simulink model "MotoSimpleECU"  (R2026b)
settings: Solver=VariableStepAuto
undefined symbols (not defined in the file): CtrlEcuRevLim, DiscIntNeverNeededParam, PlntEngTqMax
libraries: simulink x1
settings Model: Creator=The MathWorks, Inc.  LastModifiedBy=The MathWorks, Inc.

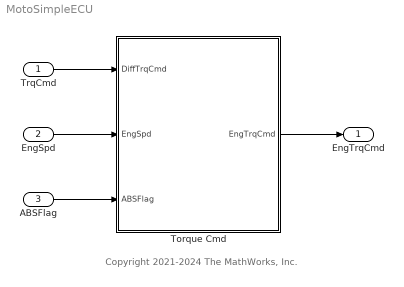
== system MotoSimpleECU ==
  note: Copyright 2021-2024 The MathWorks, Inc.
  TrqCmd : Inport
  EngSpd : Inport  Port=2
  ABSFlag : Inport  Port=3
  Torque Cmd : Subsystem  TreatAsAtomicUnit=on  SystemSampleTime=.01
  EngTrqCmd : Outport  VectorParamsAs1DForOutWhenUnconnected=off
  wires:
  ABSFlag/1 -> Torque Cmd/3(ABSFlag)
  Torque Cmd/1(EngTrqCmd) -> EngTrqCmd/1
  TrqCmd/1 -> Torque Cmd/1(DiffTrqCmd)
  EngSpd/1 -> Torque Cmd/2(EngSpd)

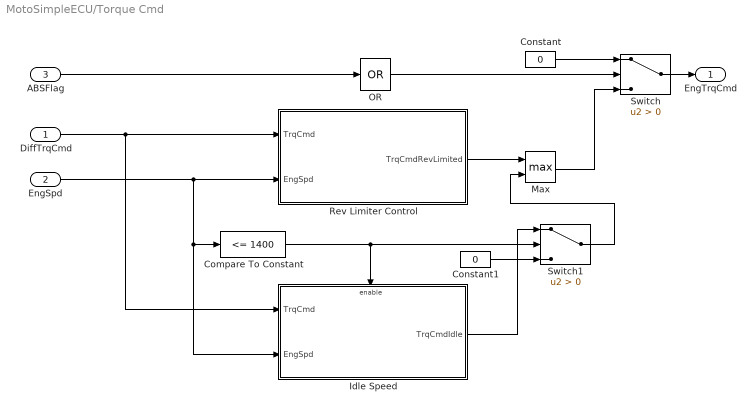
== system MotoSimpleECU/Torque Cmd ==
  DiffTrqCmd : Inport
  EngSpd : Inport  Port=2  Unit=rpm
  ABSFlag : Inport  Port=3
  Compare To Constant : simulink/Logic and Bit Operations/Compare To Constant  relop=<=  const=1400  OutDataTypeStr=boolean  ZeroCross=off
  Constant : Constant  Value=0
  Constant1 : Constant  Value=0
  Idle Speed : Subsystem
  Max : MinMax  Function=max  Inputs=2
  OR : Logic  Operator=OR  Inputs=1  AllPortsSameDT=off  OutDataTypeStr=boolean
  Rev Limiter Control : Subsystem
  Switch : Switch  Criteria=u2 > Threshold  ZeroCross=off  SaturateOnIntegerOverflow=off  InputSameDT=off
  Switch1 : Switch  Criteria=u2 > Threshold  ZeroCross=off  SaturateOnIntegerOverflow=off  InputSameDT=off
  EngTrqCmd : Outport
  wires:
  Switch1/1 -> Max/2
  Constant1/1 -> Switch1/3
  Compare To Constant/1 -> Switch1/2, Idle Speed/Enable
  Idle Speed/1(TrqCmdIdle) -> Switch1/1
  Rev Limiter Control/1(TrqCmdRevLimited) -> Max/1
  DiffTrqCmd/1 -> Rev Limiter Control/1(TrqCmd), Idle Speed/1(TrqCmd)
  EngSpd/1 -> Rev Limiter Control/2(EngSpd), Compare To Constant/1, Idle Speed/2(EngSpd)
  Max/1 -> Switch/3
  Switch/1 -> EngTrqCmd/1
  ABSFlag/1 -> OR/1
  Constant/1 -> Switch/1
  OR/1 -> Switch/2

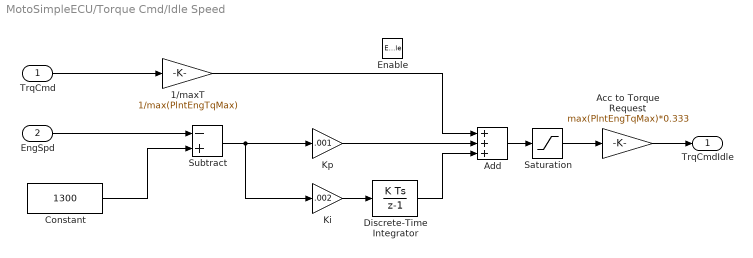
== system MotoSimpleECU/Torque Cmd/Idle Speed ==
  TrqCmd : Inport
  EngSpd : Inport  Port=2
  Enable : EnablePort  StatesWhenEnabling=reset  ZeroCross=off
  1/maxT : Gain  Gain=1/max(PlntEngTqMax)
  Acc to Torque Request : Gain  Gain=max(PlntEngTqMax)*0.333
  Add : Sum  Inputs=+++
  Constant : Constant  Value=1300  SampleTime=-1
  Discrete-Time Integrator : DiscreteIntegrator  SampleTime=-1  LimitOutput=on  UpperSaturationLimit=1  LowerSaturationLimit=0  ICPrevOutput=DiscIntNeverNeededParam  ICPrevScaledInput=DiscIntNeverNeededParam
  Ki : Gain  Gain=.002
  Kp : Gain  Gain=.001
  Saturation : Saturate  UpperLimit=1  LowerLimit=0  ZeroCross=off
  Subtract : Sum  Inputs=-+
  TrqCmdIdle : Outport  VectorParamsAs1DForOutWhenUnconnected=off
  wires:
  1/maxT/1 -> Add/1
  Saturation/1 -> Acc to Torque Request/1
  Acc to Torque Request/1 -> TrqCmdIdle/1
  Ki/1 -> Discrete-Time Integrator/1
  Kp/1 -> Add/2
  Subtract/1 -> Kp/1, Ki/1
  Discrete-Time Integrator/1 -> Add/3
  Constant/1 -> Subtract/2
  TrqCmd/1 -> 1/maxT/1
  Add/1 -> Saturation/1
  EngSpd/1 -> Subtract/1

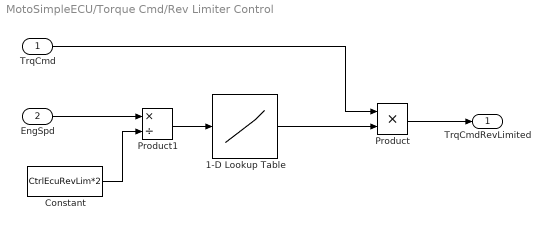
== system MotoSimpleECU/Torque Cmd/Rev Limiter Control ==
  TrqCmd : Inport
  EngSpd : Inport  Port=2
  1-D Lookup Table : Lookup_n-D  NumberOfTableDimensions=1  BreakpointsForDimension1=[1 1.01]  Table=[1 0]  ExtrapMethod=Clip  InternalRulePriority=Speed  RndMeth=Simplest
  Constant : Constant  Value=CtrlEcuRevLim*2
  Product : Product
  Product1 : Product  Inputs=*/
  TrqCmdRevLimited : Outport  VectorParamsAs1DForOutWhenUnconnected=off
  wires:
  EngSpd/1 -> Product1/1
  Product/1 -> TrqCmdRevLimited/1
  1-D Lookup Table/1 -> Product/2
  TrqCmd/1 -> Product/1
  Constant/1 -> Product1/2
  Product1/1 -> 1-D Lookup Table/1
